simulink model "OpenLoop"  (R2017b)
settings: Solver=VariableStepAuto  StartTime=0.0  StopTime=10.0  RelTol=1e-3
undefined symbols (not defined in the file or in its folder): J_l, J_m, Ke, Kt, L, N, r, R, Tf
settings Model: Creator=dp27349  LastModifiedBy=dp27349

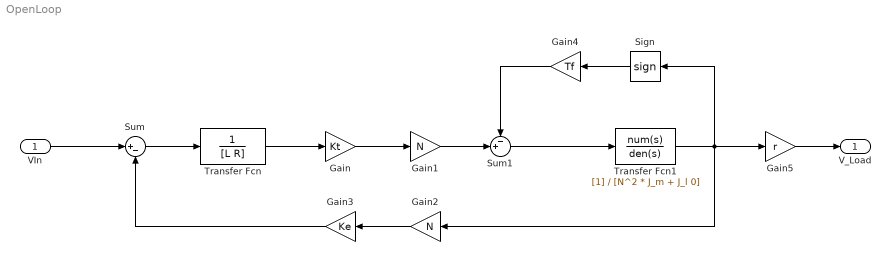
== system OpenLoop ==
  VIn : Inport
  Gain : Gain  Gain=Kt
  Gain1 : Gain  Gain=N
  Gain2 : Gain  Gain=N
  Gain3 : Gain  Gain=Ke
  Gain4 : Gain  Gain=Tf
  Gain5 : Gain  Gain=r
  Sign : Signum
  Sum : Sum  Inputs=|+-
  Sum1 : Sum  Inputs=-+|
  Transfer Fcn : TransferFcn  Denominator=[L R]
  Transfer Fcn1 : TransferFcn  Denominator=[N^2 * J_m + J_l 0]
  V_Load : Outport
  wires:
  Sum/1 -> Transfer Fcn/1
  Transfer Fcn/1 -> Gain/1
  Gain/1 -> Gain1/1
  Gain1/1 -> Sum1/2
  Sum1/1 -> Transfer Fcn1/1
  Gain2/1 -> Gain3/1
  Transfer Fcn1/1 -> Gain5/1, Gain2/1, Sign/1
  Gain3/1 -> Sum/2
  Sign/1 -> Gain4/1
  Gain4/1 -> Sum1/1
  VIn/1 -> Sum/1
  Gain5/1 -> V_Load/1
